simulink model "Lab4"  (R2016b)
settings: Solver=ode3  StartTime=0.0  StopTime=10  FixedStep=5e-6  RelTol=1e-5  EnableMultiTasking=on
libraries: commfilt2 x2, commchan3 x1, commsink2 x1, commrandsrc2 x1
settings Model: Creator=Dennis Silage  LastModifiedBy=avile
settings DataIOCC: LimitDataPoints=on  SaveFormat=Array  SignalLoggingSaveFormat=ModelDataLogs
settings OptimizationCC: ExpressionDepthLimit=2147483647  InitFltsAndDblsToZero=on  LifeSpan=inf
settings DebuggingCC: UnderspecifiedInitializationDetection=Classic  MergeDetectMultiDrivingBlocksExec=none  FcnCallInpInsideContextMsg=warning  StateNameClashWarn=warning  SFUnexpectedBacktrackingDiag=warning  SFNoUnconditionalDefaultTransitionDiag=warning  SFExecutionAtInitializationDiag=none
settings HardwareCC: ProdBitPerPointer=32  ProdBitPerSizeT=32  ProdBitPerPtrDiffT=32  ProdLargestAtomicFloat=None  ProdIntDivRoundTo=Undefined  ProdEndianess=Unspecified  ProdWordSize=32  ProdHWDeviceType=32-bit Generic
settings ModelReferenceCC: PropagateSignalLabelsOutOfModel=off
settings GRTTargetCC: TargetLangStandard=C89/C90 (ANSI)  GeneratePreprocessorConditionals=Disable all  CombineOutputUpdateFcns=off  GRTInterface=on
settings ConfigComp: CovMetricSettings=dw  CovHtmlReporting=on  CovSaveCumulativeToWorkspaceVar=on  CovSaveSingleToWorkspaceVar=on  CovExternalEMLEnable=off  CovSFcnEnable=off

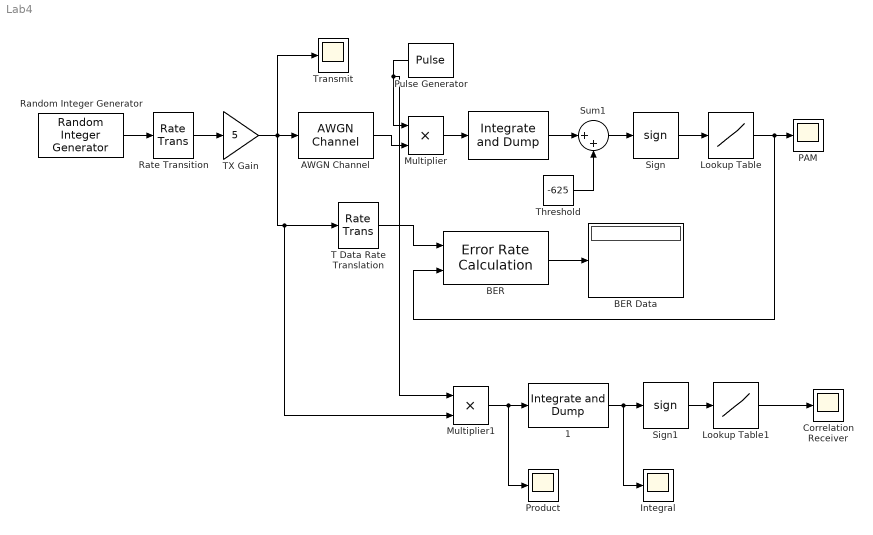
== system Lab4 ==
  " " : commfilt2/Integrate and Dump  obssamples=50  offsetsamples=0  nodump=off  roundingMode=Floor  overflowMode=off  outputDataTypeStr=Inherit: Same as accumulator  outputLastDataTypeStr=Inherit: Same as accumulator
  " 1" : commfilt2/Integrate and Dump  obssamples=50  offsetsamples=0  nodump=off  roundingMode=Floor  overflowMode=off  outputDataTypeStr=Inherit: Same as accumulator  outputLastDataTypeStr=Inherit: Same as accumulator
  AWGN Channel : commchan3/AWGN Channel  InputProcessing=Inherited (this choice will be removed - see release notes)  seed=randseed  noiseMode="Signal to noise ratio  (Eb/No)"  EbNodB=40  EsNodB=10  SNRdB=10  bitsPerSym=1  Ps=25  Tsym=1e-3  variance=0
  BER : commsink2/Error Rate Calculation  N=1  st_delay=0  cp_mode=Entire frame  subframe=[]  PMode=Port  WsName=ErrorVec  RsMode2=off  stop=off  numErr=100  maxBits=1e6
  BER Data : Display
  Correlation Receiver : Scope
  Integral : Scope
  Lookup Table : Lookup_n-D  NumberOfTableDimensions=1  BreakpointsForDimension1=[-1, 0, 1]  Table=[0, 0, 5]  InternalRulePriority=Speed  RndMeth=Nearest  InputSameDT=on
  Lookup Table1 : Lookup  InputValues=[-1,0,1]  Table=[-1,-1,1]
  Multiplier : Product  RndMeth=Zero
  Multiplier1 : Product  RndMeth=Zero
  PAM : Scope
  Product : Scope
  Pulse Generator : DiscretePulseGenerator  PulseType=Time based  Amplitude=12  Period=250e-6  PulseWidth=30  PhaseDelay=125e-6
  Random Integer Generator : commrandsrc2/Random Integer Generator  mul=2  seed=randseed  Ts=1e-3  frameBased=off  sampPerFrame=50  orient=on  outDataType=double
  Rate Transition : RateTransition  OutPortSampleTime=5e-6
  Sign : Signum
  Sign1 : Signum
  Sum1 : Sum  Inputs=|++
  T Data Rate Translation : RateTransition  OutPortSampleTime=25e-5
  TX Gain : Gain  Gain=5
  Threshold : Constant  Value=-625
  Transmit : Scope
  wires:
  TX Gain/1 -> Multiplier1/2, T Data Rate Translation/1, AWGN Channel/1, Transmit/1
  Random Integer Generator/1 -> Rate Transition/1
  BER/1 -> BER Data/1
  T Data Rate Translation/1 -> BER/1
  Multiplier/1 -> " "/1
  Pulse Generator/1 -> Multiplier1/1, Multiplier/1
  Rate Transition/1 -> TX Gain/1
  Threshold/1 -> Sum1/2
  Sum1/1 -> Sign/1
  " "/1 -> Sum1/1
  Sign/1 -> Lookup Table/1
  Lookup Table/1 -> BER/2, PAM/1
  AWGN Channel/1 -> Multiplier/2
  Multiplier1/1 -> " 1"/1, Product/1
  Sign1/1 -> Lookup Table1/1
  " 1"/1 -> Sign1/1, Integral/1
  Lookup Table1/1 -> Correlation Receiver/1
